simulink model "Ctrls_Software_Strong_Arm"  (R2018a)
settings: Solver=FixedStepAuto  StartTime=0.0  StopTime=10.0  FixedStep=Ts  RelTol=1e-3  EnableMultiTasking=on
values from neighbouring files (symbols this model uses):
  Ts = .001    (= 0.001)    [Setup_Strong_Arm_Parameters.m]
libraries: arduinolib x4, dspsigops x1
settings Model: ExtModeTrigDuration=2  Creator=dtmasetti  LastModifiedBy=dtmasetti
settings OptimizationCC: EnhancedBackFolding=on  PassReuseOutputArgsThreshold=0  MaxStackSize=64  OptimizeBlockOrder=speed  DifferentSizesBufferReuse=on  OptimizationCustomize=off
settings DebuggingCC: ParameterTunabilityLossMsg=error
settings HardwareCC: ProdBitPerInt=16  ProdBitPerPointer=16  ProdBitPerSizeT=16  ProdBitPerPtrDiffT=16  ProdLargestAtomicFloat=None  ProdWordSize=8  ProdHWDeviceType=Atmel->AVR  UseEmbeddedCoderFeatures=off
settings SFSimCC: MATLABDynamicMemAlloc=off
settings RTWCC: SystemTargetFile=ert.tlc  HardwareBoard=Arduino Mega 2560  TLCOptions=-aInlineSetEventsForThisBaseRateFcn=TLC_FALSE -aSuppressMultiTaskScheduler=TLC_FALSE -aRateBasedStepFcn=1  TemplateMakefile=ert_default_tmf  GenerateReport=on  Toolchain=Arduino AVR  BuildConfiguration=Faster Runs  LaunchReport=on
settings CodeAppCC: ForceParamTrailComments=on  OperatorAnnotations=on
settings ERTTargetCC: ERTCustomFileBanners=off  SupportContinuousTime=on  SupportNonInlinedSFcns=on  RemoveResetFunc=off  SupportVariableSizeSignals=on  ModelStepFunctionPrototypeControlCompliant=off

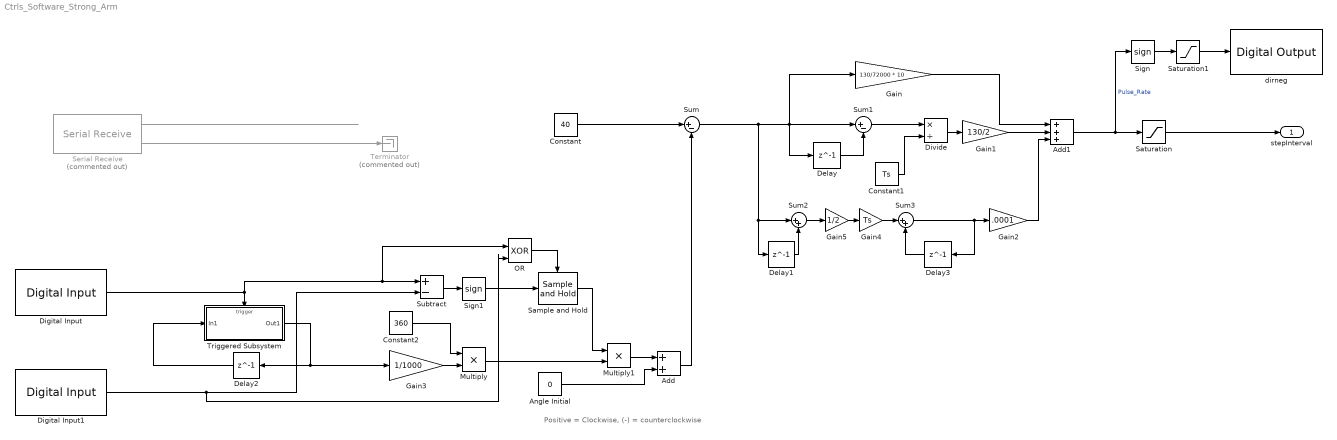
== system Ctrls_Software_Strong_Arm ==
  note: Positive = Clockwise, (-) = counterclockwise
  Add : Sum
  Add1 : Sum  Inputs=+++
  Angle Initial : Constant  Value=0
  Constant : Constant  Value=40
  Constant1 : Constant  Value=Ts
  Constant2 : Constant  Value=360
  Delay{,1..3} (4 alike) : Delay  DelayLength=1
  Digital Input : arduinolib/Digital Input  pinNumber=18  sampleTime=Ts  blockPlatform=arduino
      settings: SourceProductName=Simulink Support Package for Arduino Hardware
  Digital Input1 : arduinolib/Digital Input  pinNumber=19  sampleTime=Ts  blockPlatform=arduino
      settings: SourceProductName=Simulink Support Package for Arduino Hardware
  Divide : Product  Inputs=*/
  Gain : Gain  Gain=130/72000 * 10
  Gain1 : Gain  Gain=130/2
  Gain2 : Gain  Gain=.0001
  Gain3 : Gain  Gain=1/1000
  Gain4 : Gain  Gain=Ts
  Gain5 : Gain  Gain=1/2
  Multiply : Product
  Multiply1 : Product
  OR : Logic  Operator=XOR  IconShape=distinctive  AllPortsSameDT=off  OutDataTypeStr=boolean
  Sample and Hold : dspsigops/Sample and Hold  trig=Rising edge  initCond=0  latchinput=off
  Saturation : Saturate  UpperLimit=1000  LowerLimit=300
  Saturation1 : Saturate  UpperLimit=1  LowerLimit=0
  Serial Receive : arduinolib/Serial Receive  Commented=on  isARMArch=off  portNumber=0  DataType=uint8  Datalength=1  SampleTime=5  showOutStatus=on  blockPlatform=arduino
      settings: SourceProductName=Simulink Support Package for Arduino Hardware  SourceProductBaseCode=ARDUINO
  Sign : Signum
  Sign1 : Signum
  Subtract : Sum  Inputs=+-
  Sum : Sum  Inputs=|+-
  Sum1 : Sum  Inputs=|+-
  Sum2 : Sum  Inputs=|++
  Sum3 : Sum  Inputs=|++
  Terminator : Terminator  Commented=on
  Triggered Subsystem : Subsystem  TreatAsAtomicUnit=on
  dirneg : arduinolib/Digital Output  pinNumber=24  blockPlatform=arduino
  stepInterval : Outport
  wires:
  Serial Receive/2 -> Terminator/1
  Serial Receive/1 -> ?
  Gain/1 -> Add1/1
  Delay/1 -> Sum1/2
  Sum1/1 -> Divide/1
  Constant1/1 -> Divide/2
  Divide/1 -> Gain1/1
  Gain1/1 -> Add1/2
  Delay1/1 -> Sum2/2
  Gain2/1 -> Add1/3
  Add1/1 -> Sign/1, Saturation/1  "Pulse_Rate"
  Saturation/1 -> stepInterval/1
  Sign/1 -> Saturation1/1
  Saturation1/1 -> dirneg/1
  Angle Initial/1 -> Add/2
  Constant2/1 -> Multiply/1
  Gain3/1 -> Multiply/2
  Multiply/1 -> Multiply1/2
  Add/1 -> Sum/2
  Digital Input/1 -> OR/1, Subtract/1, Triggered Subsystem/Trigger
  Digital Input1/1 -> Subtract/2, OR/2
  Triggered Subsystem/1(Out1) -> Gain3/1, Delay2/1
  Delay2/1 -> Triggered Subsystem/1(In1)
  Subtract/1 -> Sign1/1
  Sign1/1 -> Sample and Hold/1
  OR/1 -> Sample and Hold/Trigger
  Sample and Hold/1 -> Multiply1/1
  Multiply1/1 -> Add/1
  Sum2/1 -> Gain5/1
  Sum/1 -> Sum2/1, Delay1/1, Sum1/1, Delay/1, Gain/1
  Gain4/1 -> Sum3/1
  Gain5/1 -> Gain4/1
  Sum3/1 -> Delay3/1, Gain2/1
  Delay3/1 -> Sum3/2
  Constant/1 -> Sum/1

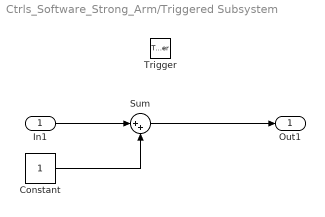
== system Ctrls_Software_Strong_Arm/Triggered Subsystem ==
  In1 : Inport
  Trigger : TriggerPort  VariantControl=Variant
  Constant : Constant
  Sum : Sum  Inputs=|++
  Out1 : Outport
  wires:
  In1/1 -> Sum/1
  Constant/1 -> Sum/2
  Sum/1 -> Out1/1
